simulink model "single_system_2021b1"  (R2021b)
settings: Solver=VariableStepAuto  StartTime=0.0  StopTime=1  RelTol=1e-3
model workspace (MAT data in the model file):
  ext_ctrl = Simulink.Parameter
  ext_ctrl.DataType = 'auto'
  ext_ctrl.Complexity = 'real'
  ext_ctrl.Dimensions = [0 0]
  ext_u_f = Simulink.Parameter
  ext_u_f.DataType = 'auto'
  ext_u_f.Complexity = 'real'
  ext_u_f.Dimensions = [0 0]
  ext_u_t = Simulink.Parameter
  ext_u_t.DataType = 'auto'
  ext_u_t.Complexity = 'real'
  ext_u_t.Dimensions = [0 0]
values from neighbouring files (symbols this model uses):
  dt = 0.01    [init_params.m]
  initial_state_x0 = Simulink.Parameter(initial_state_x0)    [init_params.m]    (also in single_model_verification_script.m = [W0; R0; dP0; P0]; team_model_conf_comp_script.m = [W0; R0; dP0; P0]; team_model_tethered_tilt.m = [W0; R0; dP0; P0]; team_model_tracking_script.m = [W0; R0; dP0; P0])
undefined symbols (not defined in the file or in its folder): ctrl_params, drone_params, env_params, initial_state_z0
libraries: dspindex x5
settings Model: Creator=NTU  LastModifiedBy=NTU
settings DataIOCC: SaveFinalState=on  SaveState=on
settings DebuggingCC: UnconnectedInputMsg=none  UnconnectedOutputMsg=none  UnconnectedLineMsg=none
settings ModelReferenceCC: EnableRefExpFcnMdlSchedulingChecks=off
settings RTWCC: DLArmComputeVersion=20.02.1

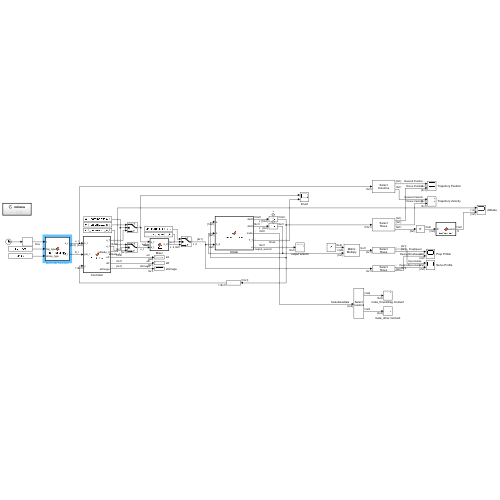
[thumbnail: Simulink's stored preview of the top-level diagram]
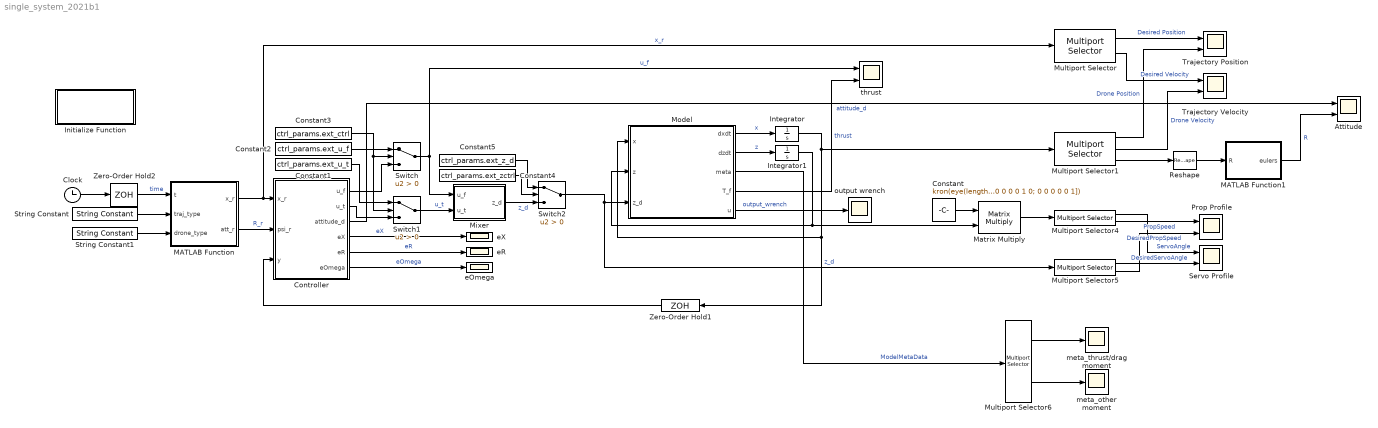
== system single_system_2021b1 ==
  Attitude : Scope  NumInputPorts=2
  Clock : Clock
  Constant : Constant  Value=kron(eye(length(drone_params.psi)), [1 0 0 0 0 0;0 0 1 0 0 0; 0 0 0 0 1 0; 0 0 0 0 0 1])  VectorParams1D=off
  Constant1 : Constant  Value=ctrl_params.ext_u_t  VectorParams1D=off
  Constant2 : Constant  Value=ctrl_params.ext_u_f  VectorParams1D=off
  Constant3 : Constant  Value=ctrl_params.ext_ctrl  VectorParams1D=off
  Constant4 : Constant  Value=ctrl_params.ext_zctrl  VectorParams1D=off
  Constant5 : Constant  Value=ctrl_params.ext_z_d  VectorParams1D=off
  Controller : MATLAB Function  TreatAsAtomicUnit=on
  Initialize Function : Subsystem  TreatAsAtomicUnit=on
  Integrator : Integrator  InitialCondition=zeros([18 1])  ContinuousStateAttributes='x'
  Integrator1 : Integrator  InitialCondition=zeros([6*length(drone_params.psi) 1])  ContinuousStateAttributes='z'
  MATLAB Function : MATLAB Function  TreatAsAtomicUnit=on
  MATLAB Function1 : MATLAB Function  TreatAsAtomicUnit=on
  Matrix Multiply : Product  Multiplication=Matrix(*)
  Mixer : MATLAB Function  TreatAsAtomicUnit=on
  Model : MATLAB Function  TreatAsAtomicUnit=on
  Multiport Selector : dspindex/Multiport Selector  rowsOrCols=Columns  idxCellArray={ 1, 2 }  idxErrMode=Clip Index
  Multiport Selector1 : dspindex/Multiport Selector  rowsOrCols=Rows  idxCellArray={ [16:18], [13:15], [4:12] }  idxErrMode=Clip Index
  Multiport Selector4 : dspindex/Multiport Selector  rowsOrCols=Rows  idxCellArray={ [1 2], [3 4] }  idxErrMode=Clip Index
  Multiport Selector5 : dspindex/Multiport Selector  rowsOrCols=Rows  idxCellArray={ [1 2], [3 4] }  idxErrMode=Clip Index
  Multiport Selector6 : dspindex/Multiport Selector  rowsOrCols=Columns  idxCellArray={ [1:2], [3:5]}  idxErrMode=Clip Index
  Prop Profile : Scope  NumInputPorts=2
  Reshape : Reshape  OutputDimensionality=Customize  OutputDimensions=[3,3]
  Servo Profile : Scope  NumInputPorts=2
  String Constant : StringConstant  String=traj_type
  String Constant1 : StringConstant  String="\"single\""
  Switch : Switch  Criteria=u2 > Threshold
  Switch1 : Switch  Criteria=u2 > Threshold
  Switch2 : Switch  Criteria=u2 > Threshold
  Trajectory Position : Scope  NumInputPorts=2
  Trajectory Velocity : Scope  NumInputPorts=2
  Zero-Order Hold1 : ZeroOrderHold  SampleTime=dt
  Zero-Order Hold2 : ZeroOrderHold  SampleTime=dt
  eOmega : Scope
  eR : Scope
  eX : Scope
  meta_other moment : Scope
  meta_thrust/drag moment : Scope
  output wrench : Scope
  thrust : Scope  NumInputPorts=2
  wires:
  Switch/1 -> thrust/1, Mixer/1(u_f)  "u_f"
  Switch1/1 -> Mixer/2(u_t)  "u_t"
  Switch2/1 -> Multiport Selector5/1, Model/3(z_d)  "z_d"
  Model/1(dxdt) -> Integrator/1  "x"
  Model/2(dzdt) -> Integrator1/1  "z"
  Integrator/1 -> Zero-Order Hold1/1, Model/1(x), Multiport Selector1/1
  Integrator1/1 -> Model/2(z), Matrix Multiply/2
  MATLAB Function/1(x_r) -> Multiport Selector/1, Controller/1(x_r)  "x_r"
  MATLAB Function/2(att_r) -> Controller/2(psi_r)  "R_r"
  Clock/1 -> Zero-Order Hold2/1
  Zero-Order Hold2/1 -> MATLAB Function/1(t)  "time"
  Multiport Selector1/3 -> Reshape/1
  MATLAB Function1/1(eulers) -> Attitude/2  "R"
  Reshape/1 -> MATLAB Function1/1(R)
  Multiport Selector1/1 -> Trajectory Position/2  "Drone Position"
  Multiport Selector/2 -> Trajectory Velocity/1  "Desired Velocity"
  Multiport Selector1/2 -> Trajectory Velocity/2  "Drone Velocity"
  Multiport Selector/1 -> Trajectory Position/1  "Desired Position"
  String Constant/1 -> MATLAB Function/2(traj_type)
  String Constant1/1 -> MATLAB Function/3(drone_type)
  Controller/3(attitude_d) -> Attitude/1  "attitude_d"
  Constant/1 -> Matrix Multiply/1
  Matrix Multiply/1 -> Multiport Selector4/1
  Multiport Selector4/1 -> Servo Profile/1  "ServoAngle"
  Multiport Selector5/1 -> Servo Profile/2  "DesiredServoAngle"
  Controller/4(eX) -> eX/1  "eX"
  Model/3(meta) -> Multiport Selector6/1  "ModelMetaData"
  Zero-Order Hold1/1 -> Controller/3(y)
  Model/4(T_f) -> thrust/2  "thrust"
  Model/5(u) -> output wrench/1  "output_wrench"
  Multiport Selector6/1 -> meta_thrust/drag moment/1
  Multiport Selector6/2 -> meta_other moment/1
  Multiport Selector4/2 -> Prop Profile/1  "PropSpeed"
  Multiport Selector5/2 -> Prop Profile/2  "DesiredPropSpeed"
  Controller/5(eR) -> eR/1  "eR"
  Controller/6(eOmega) -> eOmega/1  "eOmega"
  Controller/1(u_f) -> Switch/3
  Controller/2(u_t) -> Switch1/3
  Constant1/1 -> Switch1/1
  Constant2/1 -> Switch/1
  Constant3/1 -> Switch1/2, Switch/2
  Mixer/1(z_d) -> Switch2/3  "z_d"
  Constant5/1 -> Switch2/1
  Constant4/1 -> Switch2/2

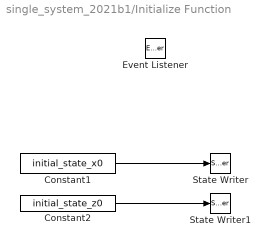
== system single_system_2021b1/Initialize Function ==
  Constant1 : Constant  Value=initial_state_x0  VectorParams1D=off
  Constant2 : Constant  Value=initial_state_z0  VectorParams1D=off
  Event Listener : EventListener  DisableCoverage=on  EventName=reset
  State Writer : StateWriter  StateOwnerBlock=../../Integrator  StateName=x
  State Writer1 : StateWriter  StateOwnerBlock=../../Integrator1  StateName=z
  wires:
  Constant1/1 -> State Writer/1
  Constant2/1 -> State Writer1/1

== matlab function single_system_2021b1/Controller ==
  settings: updateMethod=DISCRETE  sampleTime=dt
  data: u_f output; x_r input; psi_r input; y input; u_t output; attitude_d output; eX output; eR output; eOmega output; drone_params parameter; env_params parameter; ctrl_params parameter
function [u_f, u_t, attitude_d, eX, eR, eOmega] = Controller(x_r, psi_r, y, drone_params, env_params, ctrl_params)
    m = drone_params.m; % Mass, Kg
    g = env_params.g;
    I_b = drone_params.I_a + drone_params.I_fm;

    % States
    p = y(16:18);
    v = y(13:15);
    R = reshape(y(4:12), [3 3]); % 3x3
    w = y(1:3);

    % Position gain
    Kp = ctrl_params.Kp;
    Kd = ctrl_params.Kd;

    % Attitude gain
    Kr = ctrl_params.Kr;
    Ko = ctrl_params.Ko;

    eX = x_r(1:3, 1:2) - [p v];
    mu_d = x_r(1:3, 3) + Kd * (x_r(1:3, 2) - v) + Kp * (x_r(1:3, 1) - p) + [0; 0; g];

    %eX = mu_d;
    %psi_r = traj(4, 1);

    % Trajectory control
    %u_f = mu_d' * R(1:3, 3);
    u_vf = R' * mu_d;
    u_f = u_vf(3) * m;
    z_B_d = mu_d / norm(mu_d);
    x_C_d = [cos(psi_r); sin(psi_r); 0];
    cross_z_x = cross(z_B_d, x_C_d);
    y_B_d = cross_z_x / norm(cross_z_x);
    x_B_d = cross(y_B_d, z_B_d);

    R_d = [x_B_d y_B_d z_B_d];
    attitude_d = rot2zxy(R_d);

    % Attitude error
    %eRx = 0.5 * (R_d' * R - R' * R_d);
    %eR = [eRx(2, 3); eRx(3, 1); eRx(1, 2)];
    %eOmega = 0 - w;

    % Attitude control
    %Kr = diag([0.25 1 1]) * 0.1 * 2;
    %Ko = diag([0.25 1 1]) * 0.05 * 2;
    %M_d =- Kr * eR - Ko * eOmega;

    eRx = 0.5 * (R_d' * R - R' * R_d);
    eR = vee(eRx);
    eOmega = w - 0;

    M_d = I_b * (- Kr * eR - Ko * eOmega) + cross(w, I_b * w);

    u_t = M_d;
end

function eulers = rot2zxy(R)
    %phi = asin(R(:, 3, 2)); 
    psi = atan2(-R(1, 2), R(2, 2));    
    phi = atan2(R(3, 2), sqrt(1-R(3, 2).^2));
    theta = atan2(-R(3, 1), R(3, 3));
    eulers = [psi, phi, theta];
end

== matlab function single_system_2021b1/Model ==
  settings: updateMethod=CONTINUOUS
  data: x input; dxdt output; z input; z_d input; dzdt output; env_params parameter; drone_params parameter; meta output; T_f output; u output
function [dxdt, dzdt, meta, T_f, u] = system_model(x, z, z_d, env_params, drone_params)
%    [dxdt, dzdt] = tvmd_model(x, z, z_d, env_params, drone_params);
%    meta = zeros([3 5]);
%    T_f = [0;0;0];
%    thrust = 0;
   %[dxdt, dzdt, meta, T_f, u] = single_model(x, z, z_d, env_params, drone_params);
   %[dxdt, dzdt, meta, T_f, u] = single_model_RNEA(x, z, z_d, env_params, drone_params);
   %[dxdt, dzdt, meta, T_f, u] = single_model_RNEA_simplified(x, z, z_d, env_params, drone_params);
   [dxdt, dzdt, meta, T_f, u] = single_model_RNEA_full(x, z, z_d, env_params, drone_params);
   %[dxdt, dzdt, meta, T_f, u] = single_model_RNEA_simplified_full(x, z, z_d, env_params, drone_params);
end

== matlab function single_system_2021b1/Mixer ==
  settings: updateMethod=DISCRETE  sampleTime=dt
  data: u_f input; u_t input; z_d output; drone_params parameter; env_params parameter
function z_d = mixer(u_f, u_t, drone_params, env_params)
    m = drone_params.m; % Mass, Kg
    rho = env_params.rho; % kg/m3
    prop_d = env_params.prop_d; % 8 inch = 20.3 cm
    beta_allo = drone_params.beta_allo;

    r_pg = drone_params.r_pg; % Leverage length from c.p. to c.g.
    l = r_pg(3);

    CT_u = env_params.CT_u; % upper propeller thrust coefficient
    CT_l = env_params.CT_l; % lower propeller thrust coefficient
    CP_u = env_params.CP_u; % upper propeller drag coefficient
    CP_l = env_params.CP_l; % lower propeller drag coefficient

    %M_d = sat(u_t, [-1; -1; -1], [1; 1; 1]);

    % Control allocator
    Tf = u_f;
    Td = u_t(3);

    % To avoid the emergence of imaginary part
    if Tf < 0
        Tf = 0;
    end

    % To ensure the existence of inversion
    %if abs(Td) > prop_d * CP_u / CT_u * Tf
    %    Td = prop_d * CP_u / CT_u * Tf * sign(Td);
    %end

    % To prevent complex propeller speed
    Td = sat(Td, -prop_d*Tf*CP_u/CT_u, prop_d*Tf*CP_u/CT_u);

    A = [l*Tf Td; -Td l*Tf];
    eta = A \ [u_t(1); u_t(2)];

    %% Motor commands
    w_m = sqrt(beta_allo \ [Tf; Td] / (rho * prop_d^4));

    z_d = [eta; w_m];
end

== matlab function single_system_2021b1/MATLAB Function ==
  settings: updateMethod=DISCRETE  sampleTime=dt
  data: t input; x_r output; att_r output; traj_type input; drone_type input; traj_params parameter
function [x_r, att_r] = gen_trajectory(t, traj_type, drone_type, traj_params)
    traj_func = zeros([4 3]);
    coder.extrinsic('init_traj');
    traj_func = init_traj(t, traj_type, drone_type, traj_params);
    traj = traj_func;
    x_r = traj(1:3, :);

    if drone_type == "single"
        att_r = traj(4, 1);
    else
        att_r = traj(4, 1);
        %psi_d = traj(6, 1); phi_d = traj(5, 1); theta_d = traj(4, 1);
        %att_r = getI_R_B(psi_d, phi_d, theta_d);
    end
end

== matlab function single_system_2021b1/MATLAB Function1 ==
  data: R input; eulers output
function eulers = rotm2euler(R)
    psi = atan2(-R(1, 2), R(2, 2));    
    phi = atan2(R(3, 2), sqrt(abs(1-R(3, 2).^2)));
    theta = atan2(-R(3, 1), R(3, 3));
    eulers = [psi phi theta]';
end
